simulink model "simPIDClassical"  (R2023b)
settings: Solver=FixedStepAuto  StartTime=0.0  StopTime=initValues(2)  FixedStep=initValues(1)  RelTol=1e-3
values from neighbouring files (symbols this model uses):
  initValues = initialize()    [comparision.m]    (also in initialize.m = [T, tsim, stepValue, upperLim, lowerLim, K, tau, pert])
  Kd = 4 * ts/tp^2    (= 0.749219562955)    [cohenCoonPIDVar.m]    (also in programClassic.m = Kd/100)
  Ki = 3.33 / tp    (= 1.07419354839)    [cohenCoonPIDVar.m]    (also in programClassic.m = Ki - 0.4)
  Kp = 0.6 / ts    (= 0.333333333333)    [cohenCoonPIDVar.m]    (also in programClassic.m = Kp + 0.1)
libraries: slpidlib x1
settings Model: Creator=usuario  LastModifiedBy=usuario
settings DataIOCC: ReturnWorkspaceOutputs=off

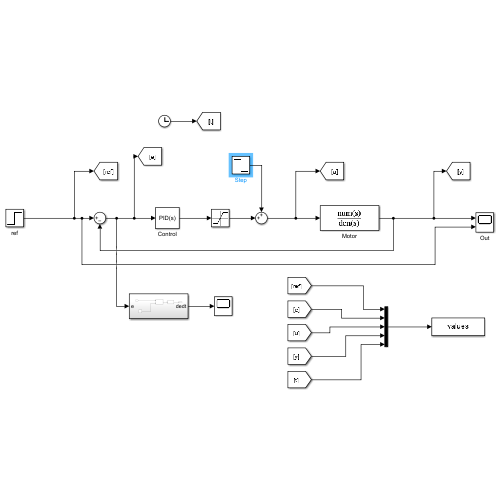
[thumbnail: Simulink's stored preview of the top-level diagram]
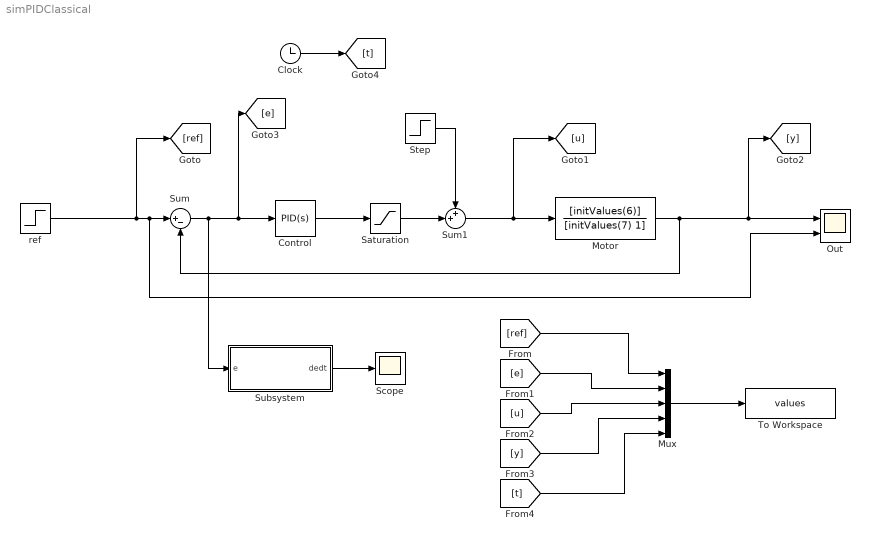
== system simPIDClassical ==
  Clock : Clock
  Control : slpidlib/PID Controller  Controller=PID  Form=Parallel  TimeDomain=Continuous-time  UseExternalTs=off  SampleTime=-1  IntegratorMethod=Forward Euler  FilterMethod=Forward Euler  ControllerParametersSource=internal  P=Kp  I=Ki  UseKiTs=off  D=Kd  N=10  UseFilter=on  TunerSelectOption=Transfer Function Based (PID Tuner App)  InitialConditionSource=internal  InitialConditionForIntegrator=0  InitialConditionForFilter=0  DifferentiatorICPrevScaledInput=0  ExternalReset=none  TrackingMode=off  Kt=1  LimitOutput=off  SatLimitsSource=internal  UpperSaturationLimit=inf  LowerSaturationLimit=-inf  LinearizeAsGain=on  AntiWindupMode=none  Kb=1  LimitIntegrator=off  UpperIntegratorSaturationLimit=inf  LowerIntegratorSaturationLimit=-inf  POutMin=[]  POutMax=[]  IOutMin=[]  IOutMax=[]  DOutMin=[]  DOutMax=[]  NOutMin=[]  NOutMax=[]  SumOutMin=[]  SumOutMax=[]  SaturationOutMin=[]  SaturationOutMax=[]  PParamMin=[]  PParamMax=[]  IParamMin=[]  IParamMax=[]  DParamMin=[]  DParamMax=[]  NParamMin=[]  NParamMax=[]  KbParamMin=[]  KbParamMax=[]  KtParamMin=[]  KtParamMax=[]  KbOutMin=[]  KbOutMax=[]  KtOutMin=[]  KtOutMax=[]  IntegratorOutMin=[]  IntegratorOutMax=[]  FilterOutMin=[]  FilterOutMax=[]  SumI1OutMin=[]  SumI1OutMax=[]  SumI2OutMin=[]  SumI2OutMax=[]  SumI3OutMin=[]  SumI3OutMax=[]  SumI4OutMin=[]  SumI4OutMax=[]  SumDOutMin=[]  SumDOutMax=[]  DifferentiatorOutMin=[]  DifferentiatorOutMax=[]  FilterDiffOutCoefMin=[]  FilterDiffOutCoefMax=[]  ReciprocalOutMin=[]  ReciprocalOutMax=[]  SumDenOutMin=[]  SumDenOutMax=[]  SumNumOutMin=[]  SumNumOutMax=[]  DivideOutMin=[]  DivideOutMax=[]  UdiffTsProdOutMin=[]  UdiffTsProdOutMax=[]  NTsProdOutMin=[]  NTsProdOutMax=[]  UintegralTsProdOutMin=[]  UintegralTsProdOutMax=[]  UngainTsProdOutMin=[]  UngainTsProdOutMax=[]  ClampingZeroOutDataTypeStr=Inherit: Inherit via back propagation  ClampingZeroOutMin=[]  ClampingZeroOutMax=[]  FilterDenConstantOutDataTypeStr=Inherit: Inherit via back propagation  FilterDenConstantOutMin=[]  FilterDenConstantOutMax=[]  PCopyOutDataTypeStr=Inherit: Inherit via back propagation  PCopyOutMin=[]  PCopyOutMax=[]  NCopyOutDataTypeStr=Inherit: Inherit via back propagation  NCopyOutMin=[]  NCopyOutMax=[]  IntegratorContinuousStateAttributes=''  IntegratorStateMustResolveToSignalObject=off  IntegratorRTWStateStorageClass=Auto  FilterContinuousStateAttributes=''  FilterStateMustResolveToSignalObject=off  FilterRTWStateStorageClass=Auto  ParallelPVariant=InternalParameters  IdealPVariant=Disabled  IVariant=InternalParameters  DVariant=InternalParameters  IntegratorVariant=Continuous  SatVariant=Disabled  AWVariant=Passthrough  PCopyVariant=Disabled  TRVariant=Disabled  FdbkBlocksVariant=Forward  IdealPFdbkVariant=Disabled  SatFdbkVariant=Disabled  DerivativeFilterVariant=ContFilter  NVariant=InternalParameters  NCopyVariant=Disabled  FilterICVariant=InternalICsFilter  IntegratorICVariant=InternalICs  ExternalResetVariant=Disabled  TRSumVariant=Passthrough  SumFdbkVariant=Disabled  SumVariant=Sum_PID  TsampFilterVariant=InternalTs  TsampNgainVariant=Passthrough  TsampIntegralVariant=Disabled_SignalSpec  ExternalSaturationOutDataTypeStr=Inherit: Same as second input
  Motor : TransferFcn  Numerator=[initValues(6)]  Denominator=[initValues(7) 1]
  Mux : Mux  Inputs=5
  Out : Scope  NumInputPorts=2
  Saturation : Saturate  UpperLimit=initValues(4)  LowerLimit=initValues(5)
  Scope : Scope
  Step : Step  Time=initValues(2)/2  After=-initValues(7)  SampleTime=0
  Subsystem : Subsystem
  Sum : Sum  Inputs=|+-
  Sum1 : Sum  Inputs=++|
  To Workspace : ToWorkspace  VariableName=values  SaveFormat=Structure  SampleTime=-1
  ref : Step  After=initValues(3)/2  SampleTime=0
  wires:
  Sum/1 -> Subsystem/1(e), Control/1, [e]
  Motor/1 -> [y], Out/1, Sum/2
  ref/1 -> [ref], Out/2, Sum/1
  [ref] -> Mux/1
  [y] -> Mux/4
  [e] -> Mux/2
  [u] -> Mux/3
  Mux/1 -> To Workspace/1
  Control/1 -> Saturation/1
  Clock/1 -> [t]
  [t] -> Mux/5
  Subsystem/1(dedt) -> Scope/1
  Saturation/1 -> Sum1/2
  Sum1/1 -> [u], Motor/1
  Step/1 -> Sum1/1

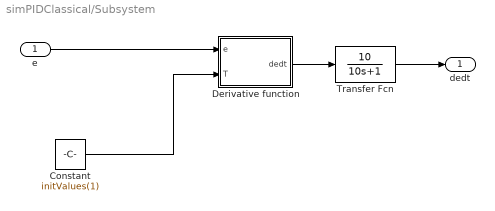
== system simPIDClassical/Subsystem ==
  e : Inport
  Constant : Constant  Value=initValues(1)
  Derivative function : MATLAB Function  TreatAsAtomicUnit=on
  Transfer Fcn : TransferFcn  Numerator=10  Denominator=[10 1]
  dedt : Outport
  wires:
  Constant/1 -> Derivative function/2(T)
  e/1 -> Derivative function/1(e)
  Derivative function/1(dedt) -> Transfer Fcn/1
  Transfer Fcn/1 -> dedt/1

== matlab function simPIDClassical/Subsystem/Derivative function ==
  settings: updateMethod=DISCRETE  sampleTime=initValues(1)
  data: e input; dedt output; T input
function dedt = fcn(e, T)
    persistent pre_e;

    if isempty(pre_e)
        pre_e = e;
    end
    
    dedt = (pre_e - e)/T;
    pre_e = e;
end
